simulink model "Exercise_1"  (R2024b)
settings: Solver=ode4  StartTime=0.0  StopTime=0.1  FixedStep=0.1  RelTol=1e-3
settings Model: Creator=Torstein  LastModifiedBy=Torstein

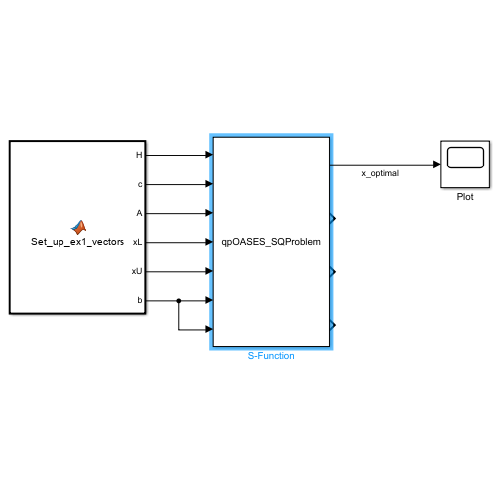
[thumbnail: Simulink's stored preview of the top-level diagram]
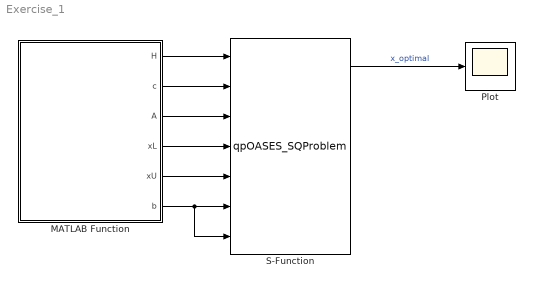
== system Exercise_1 ==
  MATLAB Function : MATLAB Function  TreatAsAtomicUnit=on
  Plot : Scope
  S-Function : S-Function  FunctionName=qpOASES_SQProblem  SFunctionDeploymentMode=off  EnableBusSupport=off
  wires:
  S-Function/1 -> Plot/1  "x_optimal"
  MATLAB Function/1(H) -> S-Function/1
  MATLAB Function/2(c) -> S-Function/2
  MATLAB Function/3(A) -> S-Function/3
  MATLAB Function/4(xL) -> S-Function/4
  MATLAB Function/5(xU) -> S-Function/5
  MATLAB Function/6(b) -> S-Function/7, S-Function/6

== matlab function Exercise_1/MATLAB Function ==
  data: H output; c output; A output; xL output; xU output; b output
function [H, c, A, xL, xU, b] = Set_up_ex1_vectors()
% Make the vectors and matixes

% Hessian matrix
H_mat = diag([6, 0, -10]);
H = H_mat(:);

% Linear term vector
c = [2.5 7 0]';

% Constraints matrix
A_mat = [2 3 4;
    -3 0 -8;
    -4 -3.2 1.8];
A = A_mat(:);

% Constraints vector
b = [5 -6 2]';

% Bounds vectors
xL = [-Inf -Inf -Inf]';
xU = [Inf Inf Inf]';
end
